simulink model "kalman"  (R2022b)
settings: Solver=FixedStepAuto  StartTime=0.0  StopTime=10.0  FixedStep=0.0001  RelTol=1e-3
values from neighbouring files (symbols this model uses):
  Ad = (eye(3)+A*Tp)    [ex6.m]    (also in kf.m)
  Bd = B*Tp    [ex6.m]    (also in kf.m)
  Cd = C    [ex6.m]    (also in kf.m)
  g = 9.81    [ex6.m]    (also in kf.m)
settings Model: Creator=MPatr  LastModifiedBy=MPatr

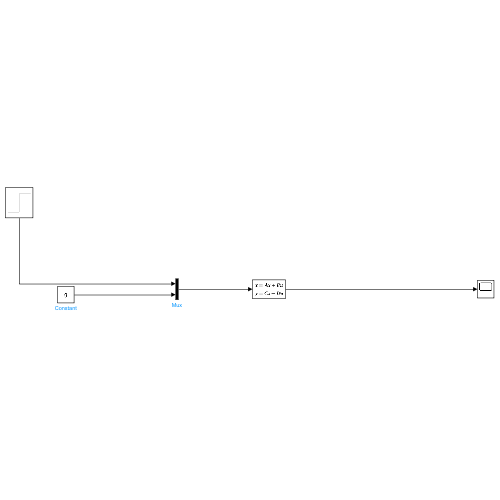
[thumbnail: Simulink's stored preview of the top-level diagram]
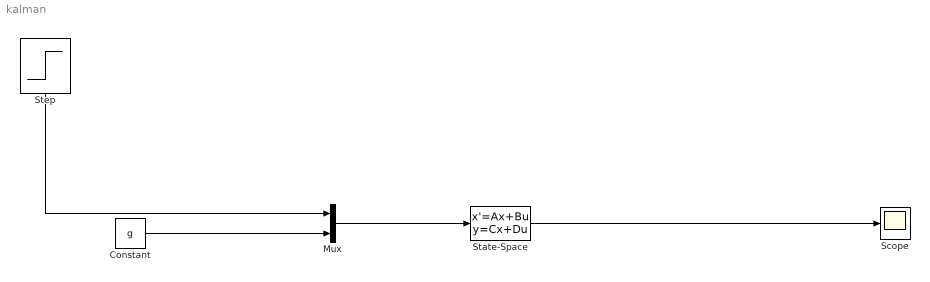
== system kalman ==
  Constant : Constant  Value=g
  Mux : Mux  Inputs=2
  Scope : Scope
  State-Space : StateSpace  A=Ad  B=Bd  C=Cd  D=[0 0]  InitialCondition=0
  Step : Step  Time=0  SampleTime=0
  wires:
  Mux/1 -> State-Space/1
  Constant/1 -> Mux/2
  Step/1 -> Mux/1
  State-Space/1 -> Scope/1
